simulink model "OFFSET_1"  (R2022b)
settings: Solver=FixedStepDiscrete  StartTime=0  StopTime=duration  FixedStep=sample_time  RelTol=1e-3
values from neighbouring files (symbols this model uses):
  LUTOFFSET =     [OFFSET_1_params.mat]
libraries: simulink x6
settings Model: Creator=Carlo_TUM  LastModifiedBy=Carlo_TUM
settings DataIOCC: LoadExternalInput=on  ReturnWorkspaceOutputs=off  ReturnWorkspaceOutputsName=off
settings OptimizationCC: DefaultParameterBehavior=Inlined  EnhancedBackFolding=on  PassReuseOutputArgsAs=Individual arguments  OptimizeBlockOrder=speed  DifferentSizesBufferReuse=on  OptimizationCustomize=off  EfficientTunableParamExpr=on
settings DebuggingCC: ParameterTunabilityLossMsg=error
settings SFSimCC: MATLABDynamicMemAlloc=off
settings RTWCC: Description=Embedded Coder  SystemTargetFile=ert.tlc  TemplateMakefile=ert_default_tmf
settings CodeAppCC: ForceParamTrailComments=on  IgnoreCustomStorageClasses=off  OperatorAnnotations=on  SimulinkDataObjDesc=on  SFDataObjDesc=on  InsertBlockDesc=on
settings ERTTargetCC: TargetLangStandard=C99 (ISO)  GenerateSampleERTMain=on  InlinedParameterPlacement=NonHierarchical  ERTCustomFileTemplate=example_file_process.tlc

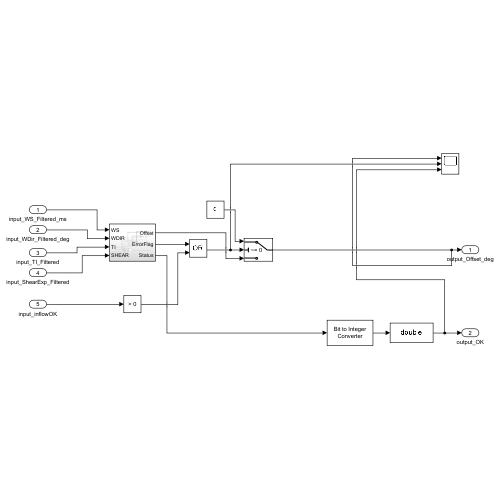
[thumbnail: Simulink's stored preview of the top-level diagram]
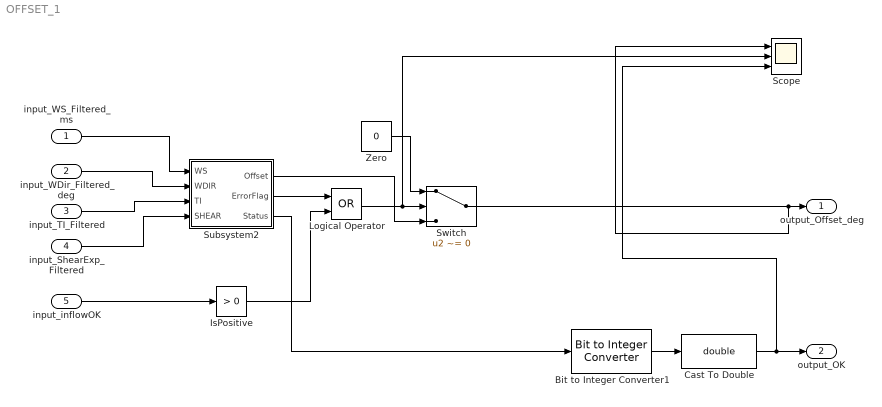
== system OFFSET_1 ==
  input_WS_Filtered_ms : Inport
  input_WDir_Filtered_deg : Inport  Port=2
  input_TI_Filtered : Inport  Port=3
  input_ShearExp_Filtered : Inport  Port=4
  input_inflowOK : Inport  Port=5
  Bit to Integer Converter1 : simulink/Logic and Bit Operations/Bit to Integer Converter  nbits=4  bitOrder=MSB first  signedOutputValues=Unsigned  outDtype=Inherit via internal rule  outDtypeSigned=Inherit via internal rule
      settings: LibrarySourceBlock=|
      | commutil2/Bit to Integer
      | Converter
  Cast To Double : DataTypeConversion  OutDataTypeStr=double  SaturateOnIntegerOverflow=off  RndMeth=Floor
  IsPositive : simulink/Logic and Bit Operations/Compare To Zero  relop=>  OutDataTypeStr=boolean
  Logical Operator : Logic  Operator=OR  AllPortsSameDT=off  OutDataTypeStr=boolean
  Scope : Scope  NumInputPorts=3
  Subsystem2 : Subsystem
  Switch : Switch  Criteria=u2 ~= 0  SaturateOnIntegerOverflow=off  InputSameDT=off
  Zero : Constant  Value=0  OutDataTypeStr=Inherit: Inherit via back propagation
  output_Offset_deg : Outport  VectorParamsAs1DForOutWhenUnconnected=off
  output_OK : Outport  Port=2  VectorParamsAs1DForOutWhenUnconnected=off
  wires:
  Cast To Double/1 -> Scope/3, output_OK/1
  Subsystem2/3(Status) -> Bit to Integer Converter1/1
  Switch/1 -> Scope/1, output_Offset_deg/1
  input_inflowOK/1 -> IsPositive/1
  Bit to Integer Converter1/1 -> Cast To Double/1
  input_TI_Filtered/1 -> Subsystem2/3(TI)
  Subsystem2/2(ErrorFlag) -> Logical Operator/1
  input_WS_Filtered_ms/1 -> Subsystem2/1(WS)
  input_WDir_Filtered_deg/1 -> Subsystem2/2(WDIR)
  IsPositive/1 -> Logical Operator/2
  Subsystem2/1(Offset) -> Switch/3
  Zero/1 -> Switch/1
  Logical Operator/1 -> Scope/2, Switch/2
  input_ShearExp_Filtered/1 -> Subsystem2/4(SHEAR)

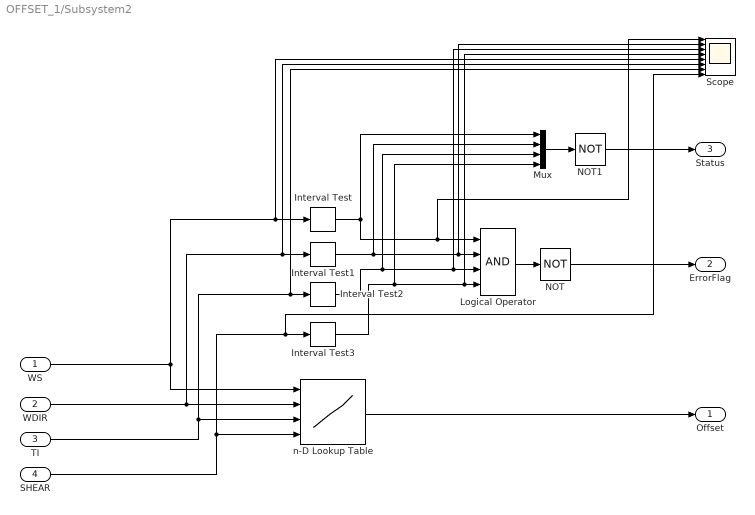
== system OFFSET_1/Subsystem2 ==
  WS : Inport
  WDIR : Inport  Port=2
  TI : Inport  Port=3
  SHEAR : Inport  Port=4
  Interval Test : simulink/Logic and Bit Operations/Interval Test  IntervalClosedRight=on  uplimit=12  IntervalClosedLeft=on  lowlimit=3  OutDataTypeStr=boolean
  Interval Test1 : simulink/Logic and Bit Operations/Interval Test  IntervalClosedRight=on  uplimit=260  IntervalClosedLeft=on  lowlimit=185  OutDataTypeStr=boolean
  Interval Test2 : simulink/Logic and Bit Operations/Interval Test  IntervalClosedRight=on  uplimit=0.4  IntervalClosedLeft=on  lowlimit=0  OutDataTypeStr=boolean
  Interval Test3 : simulink/Logic and Bit Operations/Interval Test  IntervalClosedRight=on  uplimit=0.99  IntervalClosedLeft=on  lowlimit=-0.99  OutDataTypeStr=boolean
  Logical Operator : Logic  Inputs=4  AllPortsSameDT=off  OutDataTypeStr=boolean
  Mux : Mux
  NOT : Logic  Operator=NOT  IconShape=distinctive  AllPortsSameDT=off  OutDataTypeStr=boolean
  NOT1 : Logic  Operator=NOT  IconShape=distinctive  AllPortsSameDT=off  OutDataTypeStr=boolean
  Scope : Scope  NumInputPorts=8
  n-D Lookup Table : Lookup_n-D  NumberOfTableDimensions=4  BreakpointsForDimension1=LUTOFFSET.WindSpeed  BreakpointsForDimension2=LUTOFFSET.WindDir  BreakpointsForDimension3=LUTOFFSET.TurbInt  BreakpointsForDimension4=LUTOFFSET.Shear  Table=LUTOFFSET.Offset  ExtrapMethod=Clip  UseLastTableValue=on  InternalRulePriority=Speed  RndMeth=Simplest
      settings: InputPortMap=u0,u1,u2,u3
  Offset : Outport  VectorParamsAs1DForOutWhenUnconnected=off
  ErrorFlag : Outport  Port=2  VectorParamsAs1DForOutWhenUnconnected=off
  Status : Outport  Port=3  VectorParamsAs1DForOutWhenUnconnected=off
  wires:
  Logical Operator/1 -> NOT/1
  Interval Test3/1 -> Mux/4, Scope/4, Logical Operator/4
  WS/1 -> n-D Lookup Table/1, Scope/5, Interval Test/1
  Interval Test/1 -> Mux/1, Scope/1, Logical Operator/1
  Interval Test2/1 -> Mux/3, Scope/3, Logical Operator/3
  NOT/1 -> ErrorFlag/1
  WDIR/1 -> Scope/6, Interval Test1/1, n-D Lookup Table/2
  Interval Test1/1 -> Mux/2, Scope/2, Logical Operator/2
  TI/1 -> Scope/7, Interval Test2/1, n-D Lookup Table/3
  SHEAR/1 -> Scope/8, Interval Test3/1, n-D Lookup Table/4
  n-D Lookup Table/1 -> Offset/1
  Mux/1 -> NOT1/1
  NOT1/1 -> Status/1
